simulink model "ModelBlocks"  (R2023a)
settings: Solver=FixedStepAuto  StartTime=0.0  StopTime=6  FixedStep=1e-6  RelTol=1e-15
model workspace (MAT data in the model file):
  N_p0 = 5
  N_v0 = 0
  N_w0 = 0
  t_ion = 0
  t_p = 12
  t_pump = 32
  t_release = 5
  t_retention = 2
settings Model: ParameterArgumentNames=N_p0,N_v0,N_w0,t_ion,t_p,t_pump,t_release,t_retention  Creator=levsi  LastModifiedBy=levsi
settings DataIOCC: ReturnWorkspaceOutputs=off

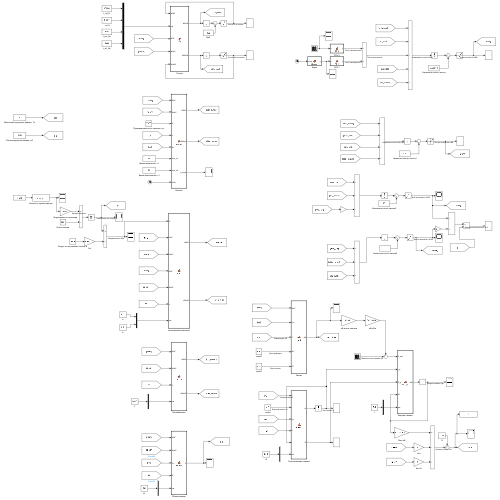
[thumbnail: Simulink's stored preview of the top-level diagram]
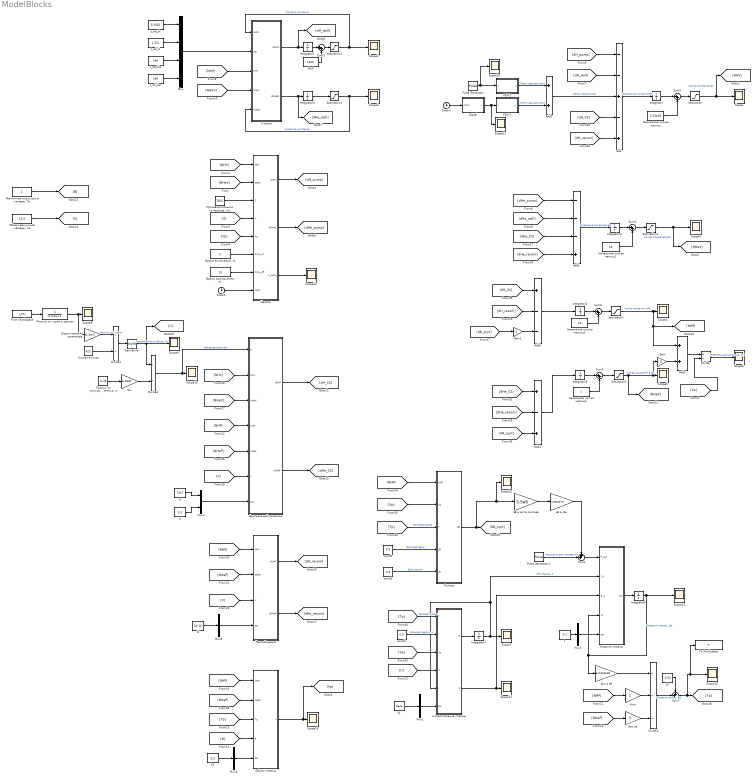
== system ModelBlocks ==
  2pi : Gain  Gain=6.2832
  Add : Sum  Inputs=--+-+
  Add1 : Sum  Inputs=---+
  Add2 : Sum
  Add3 : Sum  Inputs=+--
  Add4 : Sum  Inputs=+-+
  Add5 : Sum
  Clock1 : Clock
  Clock4 : Clock
  Derivative : Derivative
  Divide : Product  Inputs=*/
  Divide1 : Product  Inputs=*//
  Divide2 : Product  Inputs=*/
  Divide3 : Product  Inputs=*/
  From Workspace : FromWorkspace  VariableName=I_CS  OutputAfterFinalValue=Setting to zero
  Gain : Gain  Gain=2
  Gain1 : Gain  Gain=2
  H+e : Gain  Gain=2
  He+2e : Gain  Gain=3
  Integrator{,1..7} (8 alike) : Integrator  LowerSaturationLimit=0
  Mux : Mux
  Mux{1,3..5} (4 alike) : Mux  Inputs=1
  Mux2 : Mux  Inputs=2
  Nw0 : Constant  Value=1e22
  PEV-1 : MATLAB Function  TreatAsAtomicUnit=on
  PEV-3 : MATLAB Function  TreatAsAtomicUnit=on
  Pulse Generator : DiscretePulseGenerator  PulseType=Time based  Amplitude=35.8  Period=1  PulseWidth=50
  Pulse Generator1 : DiscretePulseGenerator  PulseType=Time based  Amplitude=0  Period=100  PhaseDelay=2
  Saturation{,1..5} (6 alike) : Saturate  UpperLimit=1e30  LowerLimit=0
  Scope{,1..18} (19 alike) : Scope
  Signal : MATLAB Function  TreatAsAtomicUnit=on
  Sum1 : Sum  Inputs=++|
  Sum{2..6} (5 alike) : Sum  Inputs=|++
  Sum7 : Sum  Inputs=++|
  To Workspace : ToWorkspace  VariableName=T  SaveFormat=Timeseries  SampleTime=0.00001
  a : Constant  Value=7e17
  b : Constant  Value=0.1
  b1 : Constant  Value=0.2
  const2 : Constant  Value=0.5
  const3 : Constant  Value=0.5
  const4 : Constant  Value=0.9
  t : Constant  Value=0.1
  t1 : Constant  Value=1e-16
  t2 : Constant  Value=3e-6
  t3 : Constant  Value=0.03
  t_rel_H : Constant  Value=1.331
  t_rel_He : Constant  Value=1e6
  t_ret_H : Constant  Value=0.0003
  t_ret_He : Constant  Value=1e6
  "Время включения, с1" : Constant  Value=0
  "Время выключения, с1" : Constant  Value=10
  Дж в эВ : Gain  Gain=6.2414e18
  Индуктивность соленоида : Gain  Gain=11.4e-3
  Кол-во витков : Constant  Value=423
  "Магнитная индукция в камере, Тл" : Constant
  Насосы : MATLAB Function  TreatAsAtomicUnit=on
  Начальное кол-во частиц : Constant  Value=2.25e18
  Начальное кол-во частиц1 : Constant  Value=10
  Начальное кол-во частиц2 : Constant
  Начальное кол-во частиц3 : Constant  Value=10
  "Объем вакуумной камеры, м3 " : Constant  Value=13.5
  Объем плазмы : MATLAB Function  TreatAsAtomicUnit=on
  "Производительность насосов, л/с" : Constant  Value=7600
  "Радиус по внутренней стенке, м" : Constant  Value=0.45
  Рекомбинация : MATLAB Function  TreatAsAtomicUnit=on
  Синтез : MATLAB Function  TreatAsAtomicUnit=on
  Сопротивление пламзы : MATLAB Function  TreatAsAtomicUnit=on
  Стенка : MATLAB Function  TreatAsAtomicUnit=on
  Фильтр от шума в данных : TransferFcn  Denominator=[0.02 1]
  Центральный соленоид : MATLAB Function  TreatAsAtomicUnit=on
  Энергия плазмы : MATLAB Function  TreatAsAtomicUnit=on
  эВ в Дж : Gain  Gain=1.6022e-19
  эВ в акте синтеза : Gain  Gain=3.5e6
  wires:
  Integrator/1 -> Sum2/1
  Sum2/1 -> Saturation/1
  Saturation/1 -> [NHV], Scope/1  "Кол-во атомов H в ВК"
  Saturation1/1 -> Стенка/1(NHW), Scope2/1  "Кол-во H на стенке"
  Integrator1/1 -> Sum3/1
  Sum3/1 -> Saturation1/1
  Add/1 -> Integrator/1  "Изменение кол-ва H в ВК"
  Integrator3/1 -> Saturation3/1
  Saturation3/1 -> Scope3/1, Стенка/5(NHeW)  "Кол-во He на стенке"
  Saturation4/1 -> Scope4/1, [NHeV]  "Кол-во атомов He в ВК"
  Add1/1 -> Integrator4/1  "Изменение кол-ва He в ВК"
  Add3/1 -> Integrator2/1
  Add4/1 -> Integrator5/1
  Gain/1 -> Add5/2
  Add5/1 -> Divide/1
  "Магнитная индукция в камере, Тл"/1 -> [B]
  "Объем вакуумной камеры, м3 "/1 -> [V]
  Clock1/1 -> Насосы/8(clock)
  "Время выключения, с1"/1 -> Насосы/7(time_off)
  "Время включения, с1"/1 -> Насосы/6(time_on)
  "Производительность насосов, л/с"/1 -> Насосы/3(S)
  Divide/1 -> Scope6/1  "Электронная плотность, м-3"
  Saturation2/1 -> Scope1/1, [NHP], Add5/1  "Кол-во ионов H+ в ВК"
  Saturation5/1 -> [NHeP], Gain/1, Scope5/1  "Кол-во ионов He+ в ВК"
  Начальное кол-во частиц/1 -> Sum2/2
  Nw0/1 -> Sum3/2
  Mux/1 -> Стенка/2(par)
  t_ret_H/1 -> Mux/1
  t_rel_H/1 -> Mux/2
  t_ret_He/1 -> Mux/3
  t_rel_He/1 -> Mux/4
  Add2/1 -> Add/3  "Поток газонапуска"
  PEV-3/1(y) -> Add2/1  "Поток газонапуска H"
  PEV-1/1(y) -> Add2/2  "Поток газонапуска H"
  Pulse Generator/1 -> Scope10/1, PEV-3/1(u)
  Signal/1(y) -> Scope11/1, PEV-1/1(u)
  Clock4/1 -> Signal/1(clock)
  Sum4/1 -> Saturation4/1
  Integrator4/1 -> Sum4/1
  Начальное кол-во частиц1/1 -> Sum4/2
  Integrator2/1 -> Sum6/1
  Sum6/1 -> Saturation2/1
  Начальное кол-во частиц3/1 -> Sum6/2
  Integrator5/1 -> Sum5/1
  Sum5/1 -> Saturation5/1
  Начальное кол-во частиц2/1 -> Sum5/2
  [Vp] -> Divide/2
  [V] -> Насосы/4(V)
  [Vp] -> Насосы/5(Vp)
  Насосы/1(dNHV) -> [dH_pump]
  Насосы/2(dNHeV) -> [dHe_pump]
  [dHe_pump] -> Add1/1
  [dH_pump] -> Add/1
  Насосы/3(t_pump) -> Scope12/1
  [NHeV] -> Насосы/2(NHeV)
  [NHV] -> Насосы/1(NHV)
  [dH_wall] -> Add/2
  [dHe_wall] -> Add1/2
  [NHV] -> Стенка/3(NHV)
  [NHeV] -> Стенка/4(NHeV)
  Стенка/2(dNHeW) -> [dHe_wall], Integrator3/1
  Стенка/1(dNHW) -> [dH_wall], Integrator1/1
  Derivative/1 -> Divide3/1, Scope9/1, [U]  "Напряжение по обходу, В"
  Divide2/1 -> Derivative/1
  Индуктивность соленоида/1 -> Divide2/1  "Магнитный поток"
  Кол-во витков/1 -> Divide2/2
  2pi/1 -> Divide3/2
  "Радиус по внутренней стенке, м"/1 -> 2pi/1
  Divide3/1 -> Центральный соленоид/1(E), Scope13/1  "Напряженность В/м"
  [V] -> Центральный соленоид/6(V)
  [NHeP] -> Центральный соленоид/5(NHeP)
  [NHP] -> Центральный соленоид/4(NHP)
  [NHeV] -> Центральный соленоид/3(NHeV)
  [NHV] -> Центральный соленоид/2(NHV)
  Mux2/1 -> Центральный соленоид/7(par)
  a/1 -> Mux2/1
  Центральный соленоид/1(dNHP) -> [dH_CS]
  [dH_CS] -> Add/4
  Фильтр от шума в данных/1 -> Индуктивность соленоида/1, Scope8/1
  From Workspace/1 -> Фильтр от шума в данных/1
  b/1 -> Mux2/2
  Центральный соленоид/2(dNHeP) -> [dHe_CS]
  Рекомбинация/1(dNHP) -> [dH_recom]
  Рекомбинация/2(dNHeP) -> [dHe_recom]
  [NHP] -> Рекомбинация/1(NHP)
  [NHeP] -> Рекомбинация/2(NHeP)
  [V] -> Рекомбинация/3(V)
  [dHe_recom] -> Add1/4
  [dH_recom] -> Add/5
  [Tp] -> Синтез/3(T)  "Температура эВ"
  [NHP] -> Синтез/1(NHP)
  [Vp] -> Синтез/2(Vp)
  const2/1 -> Синтез/4(dD)  "Доля дейтерия"
  const3/1 -> Синтез/5(dT)  "Доля трития"
  Синтез/1(dN) -> Scope15/1, эВ в акте синтеза/1, [dN_synt]
  [dN_synt] -> Add4/3
  [dN_synt] -> Gain1/1
  [Tp] -> Сопротивление пламзы/1(T)  "Температура эВ"
  const4/1 -> Сопротивление пламзы/2(r)  "Большой радиус, м"
  [Vp] -> Сопротивление пламзы/3(Vp)
  t/1 -> Mux3/1
  эВ в акте синтеза/1 -> эВ в Дж/1
  t1/1 -> Mux5/1
  Mux5/1 -> Рекомбинация/4(par)
  [dHe_CS] -> Add1/3
  [dHe_recom] -> Add4/2
  [dHe_CS] -> Add4/1
  эВ в Дж/1 -> Sum1/1
  Gain1/1 -> Add3/3
  [dH_recom] -> Add3/2
  [dH_CS] -> Add3/1
  [U] -> Сопротивление пламзы/4(U)
  Сопротивление пламзы/1(dI) -> Integrator7/1
  Integrator7/1 -> Scope7/1, Энергия плазмы/2(I_p), Сопротивление пламзы/5(I)  "Ток плазмы, А"
  t2/1 -> Mux1/1
  Mux1/1 -> Сопротивление пламзы/6(par)
  Сопротивление пламзы/2(R) -> Энергия плазмы/3(R_p), Scope17/1
  Pulse Generator1/1 -> Sum1/2  "Мощность доп нагрева, Вт"
  Integrator6/1 -> Дж в эВ/1, Энергия плазмы/4(W), Scope14/1  "Энергия плазмы, Дж"
  Энергия плазмы/1(dW) -> Integrator6/1
  Sum1/1 -> Энергия плазмы/1(P_aux)
  Mux3/1 -> Энергия плазмы/5(par)
  [NHP] -> H+e/1
  [NHeP] -> He+2e/1
  Дж в эВ/1 -> Divide1/1
  H+e/1 -> Divide1/2
  He+2e/1 -> Divide1/3
  Divide1/1 -> Sum7/2  "Энергия частиц, эВ"
  Sum7/1 -> To Workspace/1, Scope16/1, [Tp]
  t3/1 -> Sum7/1
  [B] -> Объем плазмы/4(B)
  b1/1 -> Mux4/1
  Mux4/1 -> Объем плазмы/5(par)
  [Tp] -> Объем плазмы/3(Tp)
  [NHeP] -> Объем плазмы/2(NHeP)
  [NHP] -> Объем плазмы/1(NHP)
  Объем плазмы/1(V) -> [Vp], Scope18/1

== matlab function ModelBlocks/Стенка ==
  data: dNHW output; NHW input; par input; NHV input; NHeV input; dNHeW output; NHeW input
function [dNHW, dNHeW]= wall(NHW, par, NHV, NHeV, NHeW)

%% Константы
t_retention_H = par(1); %постоянная времени поглощения H
t_release_H = par(2); %постоянная времени выхода H
t_retention_He = par(3); %постоянная времени поглощения He
t_release_He = par(4); %постоянная времени выхода He

%%
dNHW = NHV / t_retention_H - NHW / t_release_H;
dNHeW = NHeV / t_retention_He - NHeW / t_release_He;

end

== matlab function ModelBlocks/Рекомбинация ==
  data: dNHP output; dNHeP output; NHP input; NHeP input; V input; par input
function [dNHP, dNHeP] = recom(NHP, NHeP, V, par)

q = par(1);

dNHP = q * (NHP/V) * (NHP + 2 * NHeP);
dNHeP = q * (NHeP/V) * (NHP + 2 * NHeP);

end

== matlab function ModelBlocks/Центральный соленоид ==
  data: E input; NHV input; NHeV input; NHP input; NHeP input; V input; par input; dNHP output; dNHeP output
function [dNHP, dNHeP] = CS(E, NHV, NHeV, NHP, NHeP, V, par)

    %Константы и параметры
    a = par(1);
    b = par(2);
    e = 1.6022e-19; %заряд электрона, Кл
    m = 9.1094e-31; %масса электрона, кг
  
    %Расчет
    E = abs(E);
    n = (NHV + NHeV + NHP + NHeP) / V; %концентрация ядер м-3
    l = a / n; %длина свободного пробега электрона, м
    W1 = E * l; %энергия, которую преобрел электрон за длину свободного пробега, эВ
    W2 = e * E * l; %энергия, которую преобрел электрон за длину свободного пробега, Дж
    
    if W1>0
        q = (1e-19)*((2.9e3)/(W1) * exp(-15/sqrt(W1))); %сечение ионизации, м2
        nH = NHV/V; %концентрация H, м-3
        nHe = NHeV/V; %концентрация He, м-3
        ne = (NHP + NHeP)/V; %концентрация e, м-3
        ve = sqrt(2 * W2 / m);% скорость е, м/с
    else
        q = 0;
        nH = 0;
        nHe = 0;
        ne = 0;
        ve = 0;
    end

    dNHP = nH * ne * ve * q * V;
    dNHeP = nHe * ne * ve * q * b * V;

end

== matlab function ModelBlocks/Синтез ==
  data: dN output; NHP input; Vp input; T input; dD input; dT input
function dN  = synt(NHP, Vp, T, dD, dT)

%Константы
mD = 3.3436e-27; %масса дейтрона, кг
mT = 5.0072e-27; %масса тритона, кг
e = 1.6022e-19; %заряд электрона, Кл

%Расчет
vD =  sqrt(2 * (T * e) / mD); %скорость ядер Дейтерия, м/с
vT =  sqrt(2 * (T * e) /  mT); %скорость ядер Трития, м/с
v = (vD + vT) / 2; %средняя скорость ядер
T = T/1000; %Температура плазмы, кэВ
q = 2e-4/T * exp(-46/sqrt(T)); %сечение реакции DT, барн
q = q * 1e-28; %сечение реакции DT, м2

dN = q * (dD*NHP) * (dT*NHP) * v / Vp; %скорость реакции в объеме плазмы

end

== matlab function ModelBlocks/Сопротивление пламзы ==
  data: dI output; T input; r input; Vp input; R output; U input; I input; par input
function [dI, R]= current(T, r, Vp, U, I, par)

%Параметры
L = par(1); %индуктивность плазмы, Гн

%Расчет
T = T / 1000; %температура кэВ
p = 2.4e-2/(T^(3/2)); %удельное сопротивление плазмы, мкОм мм2 м-1
p = p * 1e-6 / (1000 * 1000); %удельное сопротивление плазмы, Ом м2 м-1

l = 2 * pi * r; %длина окружности по большому радиусу, м
R = p * l * l / Vp; %сопротивление плазменного шнура, Ом

dI = (U - R*I) / L; %ток плазмы, А

end

== matlab function ModelBlocks/Энергия плазмы ==
  data: dW output; P_aux input; I_p input; R_p input; W input; par input
function dW  = energy(P_aux, I_p, R_p, W, par)

%Параметры и константы
t_e = par(1);

%Расчет
P_current = R_p * I_p^2; %мощность омического нагрева, Вт
dW = P_current + P_aux - W/t_e;

end

== matlab function ModelBlocks/Signal ==
  data: clock input; y output
function y = Signal(clock)
    if clock<2.1
    y = 0;
    elseif clock<2.3
        y = 48;
    elseif clock<2.5
        y = 50;
    elseif clock<3
        y = 45;
    else
        y = 0;
    end

== matlab function ModelBlocks/Объем плазмы ==
  data: V output; NHP input; NHeP input; Tp input; B input; par input
function V  = volume(NHP, NHeP, Tp, B, par)

%Параметры и константы
b = par(1); %параметр бетта
k = 1.3806e-23; %постоянная Больцмана

%Расчет
N = NHP + NHeP; %Кол-во ядер в плазме
T = Tp * 11640; %температура плазмы, К;
P = 0.4 * B^2 * 1e6; %давление магнитного поля, Па
V = N * k * T / b / P;

end

== matlab function ModelBlocks/Насосы ==
  data: NHV input; NHeV input; S input; dNHV output; V input; Vp input; time_on input; time_off input; clock input; dNHeV output; t_pump output
function [dNHV, dNHeV, t_pump] = pump(NHV, NHeV, S, V, Vp, time_on, time_off, clock)

t_pump = (V-Vp) * 1000 / S;

if clock > time_on && clock < time_off
    dNHV = NHV / t_pump;
    dNHeV = NHeV / t_pump;
else
    dNHV = 0;
    dNHeV = 0;
end

end

== matlab function ModelBlocks/PEV-1 ==
  data: u input; y output
function y = PEV(u)
    y_vals = [0, 18, 28, 42, 62, 80, 100, 123, 154, 180, 200, 232, 259, 280, 300, 323, 346, 360, 400, 433, 450, 478, 500, 538, 552, 580, 600, 635, 668, 700, 729, 750, 770, 800, 839, 870, 900, 930, 958, 988, 1000, 1050, 1100];
    x_vals = [20, 32, 35, 40, 44.8, 48.2, 50, 52.2, 54.8, 56.5, 57.5, 60, 61.7, 62.8, 63.9, 65, 66.1, 67.5, 70, 71, 72, 74, 75, 76.5, 78, 80, 82, 83, 85, 87, 88, 90, 90.8, 91.8, 93, 94.5, 96.2, 97.2, 98, 98.2, 98.5, 98.8, 99];
    if (u >= x_vals(1))
        Gase = interp1(x_vals, y_vals, u);
    else
        Gase = 0;
    end
    y = Gase * 0.0980665*6.02e23/(60*8.31*300);
end

== matlab function ModelBlocks/PEV-3 ==
  data: u input; y output
function y = PEV(u)
    y_vals = [0, 18, 28, 42, 62, 80, 100, 123, 154, 180, 200, 232, 259, 280, 300, 323, 346, 360, 400, 433, 450, 478, 500, 538, 552, 580, 600, 635, 668, 700, 729, 750, 770, 800, 839, 870, 900, 930, 958, 988, 1000, 1050, 1100];
    x_vals = [20, 32, 35, 40, 44.8, 48.2, 50, 52.2, 54.8, 56.5, 57.5, 60, 61.7, 62.8, 63.9, 65, 66.1, 67.5, 70, 71, 72, 74, 75, 76.5, 78, 80, 82, 83, 85, 87, 88, 90, 90.8, 91.8, 93, 94.5, 96.2, 97.2, 98, 98.2, 98.5, 98.8, 99];
    if (u >= x_vals(1))
        Gase = interp1(x_vals, y_vals, u);
    else
        Gase = 0;
    end
    y = Gase * 0.0980665*6.02e23/(60*8.31*300);
end
